simulink model "Closed_Loop_Model"  (R2020a)
settings: Solver=VariableStepAuto  StartTime=0.0  StopTime=inf  RelTol=1e-3
libraries: vrlib x9, simulink x7, visionsinks x1
settings Model: Creator=Jeffrey  LastModifiedBy=seanchai

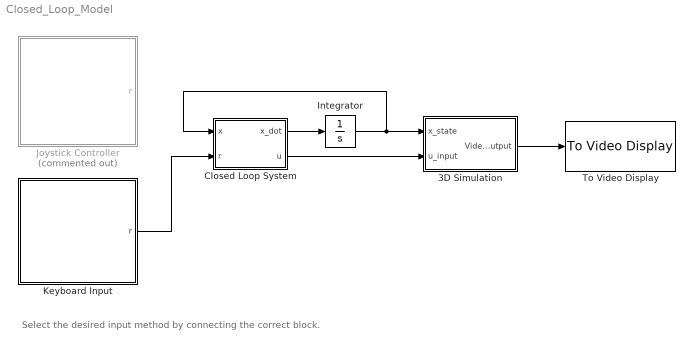
== system Closed_Loop_Model ==
  note: Select the desired input method by connecting the correct block.
  3D Simulation : Subsystem
  Closed Loop System : MATLAB Function  TreatAsAtomicUnit=on
  Integrator : Integrator  InitialCondition=[0; 0; 1; 0; 0; 0; 0; 0; 0; 0; 0; 0]
  Joystick Controller : Subsystem  Commented=on
  Keyboard Input : Subsystem
  To Video Display : visionsinks/To Video Display  windowSizeMode=Normal  openAtMdlStart=on  fullScreen=off  videoWindowX=577  videoWindowY=310  saveWindowSize=off  videoWindowWidth=640  videoWindowHeight=399  inputColorFormat=RGB  inputType=Obsolete  imagePorts=One multidimensional signal  OutputDevice=On-screen video monitor  dataOrg=Column-major  isWindowOpen=off
  wires:
  Integrator/1 -> 3D Simulation/1(x_state), Closed Loop System/1(x)
  Closed Loop System/1(x_dot) -> Integrator/1
  Closed Loop System/2(u) -> 3D Simulation/2(u_input)
  3D Simulation/1(Video Output) -> To Video Display/1
  Keyboard Input/1(r) -> Closed Loop System/2(r)

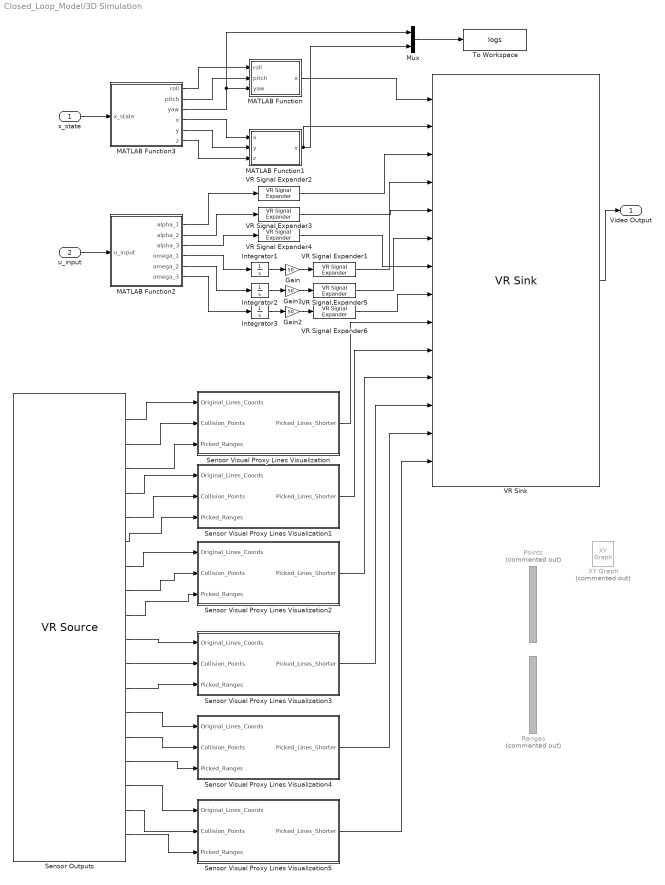
== system Closed_Loop_Model/3D Simulation ==
  x_state : Inport
  u_input : Inport  Port=2
  Gain : Gain  Gain=50
  Gain1 : Gain  Gain=50
  Gain2 : Gain  Gain=50
  Integrator1 : Integrator
  Integrator2 : Integrator
  Integrator3 : Integrator
  MATLAB Function : MATLAB Function  TreatAsAtomicUnit=on
  MATLAB Function1 : MATLAB Function  TreatAsAtomicUnit=on
  MATLAB Function2 : MATLAB Function  TreatAsAtomicUnit=on
  MATLAB Function3 : MATLAB Function  TreatAsAtomicUnit=on
  Mux : Mux  Inputs=2
  Points : Mux  Commented=on  Inputs=6
  Ranges : Mux  Commented=on  Inputs=6
  Sensor Outputs : vrlib/VR Source  InstantiateOnLoad=on  SampleTime=0.1  ViewEnable=on  RemoteChange=off  RemoteView=off  FieldsRead=Points_0006.point.61.3.1.double#PickSensor_0006.pickedPoint.60.3.1.double#PickSensor_0006.pickedRange.60.1.1.double#Points_0005.point.61.3.1.double#PickSensor_0005.pickedPoint.60.3.1.double#PickSensor_0005.pickedRange.60.1.1.double#Points_0004.point.61.3.1.double#PickSensor_0004.pickedPoint.60.3.1.double#PickSensor_0004.pickedRange.60.1.1.double#Points_0003.point.61.3.1.double#PickSensor_0003.pickedPoint.60.3.1.double#PickSensor_0003.pickedRange.60.1.1.double#Points_0002.point.61.3.1.double#PickSensor_0002.pickedPoint.60.3.1.double#PickSensor_0002.pickedRange.60.1.1.double#Points_0001.point.61.3.1.double#PickSensor_0001.pickedPoint.60.3.1.double#PickSensor_0001.pickedRange.60.1.1.double  WorldFileName=3DModel/3DModelTemplate  WorldDescription=Autonomous Airship  AutoView=on  VideoDimensions=[]  AllowVariableSize=on  FigureProperties="{'Position', 'Name', 'Viewpoint', 'CameraBound', 'CameraDirection', 'CameraPosition', 'CameraUpVector', 'ZoomFactor', 'Antialiasing', 'Headlight', 'Lighting', 'NavPanel', 'Sound', 'StatusBar', 'Stereo3D', 'Stereo3DCameraOffset', 'Stereo3DHIT', 'ToolBar', 'Textures', 'Transparency', 'Triad', 'Wireframe', 'NavZones', 'NavMode', 'NavSpeed', 'CaptureFileFormat', 'CaptureFileName', 'Record2DCompressMethod', 'Record2DCompressQuality', 'Record2D', 'Record2DFileName', 'Record2DFPS'; [1.3800000000000000e+02   1.0400000000000000e+02   5.7600000000000000e+02   3.5000000000000000e+02], 'Autonomous Airship', 'View from the Top', 'on', [0.0000000000000000e+00   0.0000000000000000e+00  -1.0000000000000000e+00], [0.0000000000000000e+00   0.0000000000000000e+00   0.0000000000000000e+00], [0.0000000000000000e+00   1.0000000000000000e+00   0.0000000000000000e+00], [1.0000000000000000e+00], 'on', 'on', 'on', 'halfbar', 'on', 'on', 'off', [1.0000000149011612e-01], [0.0000000000000000e+00], 'on', 'on', 'on', 'none', 'off', 'on', 'fly', 'normal', 'tif', '%f_anim_%n.tif', 'auto', [7.5000000000000000e+01], 'off', '%f_anim_%n.avi', 'auto'}"
      settings: SourceProductBaseCode=SL
  Sensor Visual Proxy Lines Visualization : Subsystem
  Sensor Visual Proxy Lines Visualization1 : Subsystem
  Sensor Visual Proxy Lines Visualization2 : Subsystem
  Sensor Visual Proxy Lines Visualization3 : Subsystem
  Sensor Visual Proxy Lines Visualization4 : Subsystem
  Sensor Visual Proxy Lines Visualization5 : Subsystem
  To Workspace : ToWorkspace  VariableName=logs  SampleTime=-1
      settings: Save2DSignal=2-D array (concatenate along first dimension)
  VR Signal Expander{1..6} (6 alike) : vrlib/VR Signal Expander  outwidth=4  outidx=[4]
  VR Sink : vrlib/VR Sink  InstantiateOnLoad=on  SampleTime=0.1  ViewEnable=on  RemoteChange=off  RemoteView=off  FieldsWritten=Airship.rotation.4.1.1.double#Airship.translation.3.1.1.double#Motor001.rotation.4.1.1.double#Prop001.rotation.4.1.1.double#Motor002.rotation.4.1.1.double#Prop002.rotation.4.1.1.double#Motor003.rotation.4.1.1.double#Prop003.rotation.4.1.1.double#Visual_Points_0006.point.3.-1.1.double#Visual_Points_0005.point.3.-1.1.double#Visual_Points_0004.point.3.-1.1.double#Visual_Points_0003.point.3.-1.1.double#Visual_Points_0002.point.3.-1.1.double#Visual_Points_0001.point.3.-1.1.double  WorldFileName=3DModel/3DModelTemplate.x3d  WorldDescription=Autonomous Airship  AutoView=on  VideoDimensions=[400 640]  AllowVariableSize=off  FigureProperties="{'Position', 'Name', 'Viewpoint', 'CameraBound', 'CameraDirection', 'CameraPosition', 'CameraUpVector', 'ZoomFactor', 'Antialiasing', 'Headlight', 'Lighting', 'NavPanel', 'Sound', 'StatusBar', 'Stereo3D', 'Stereo3DCameraOffset', 'Stereo3DHIT', 'ToolBar', 'Textures', 'Transparency', 'Triad', 'Wireframe', 'NavZones', 'NavMode', 'NavSpeed', 'CaptureFileFormat', 'CaptureFileName', 'Record2DCompressMethod', 'Record2DCompressQuality', 'Record2D', 'Record2DFileName', 'Record2DFPS'; [5.0000000000000000e+00   9.5000000000000000e+01   5.7600000000000000e+02   3.5000000000000000e+02], 'Autonomous Airship', 'View from the Top', 'on', [-6.0928554571654234e-02  -3.0894106635612190e-01  -9.4912756189910374e-01], [-1.3366649406455859e+00   3.5008055805870580e-01  -4.6890079737670746e+01], [-1.4625128619556730e-02   9.5106843948065223e-01  -3.0863397259001091e-01], [1.0000000000000000e+00], 'off', 'on', 'on', 'halfbar', 'on', 'on', 'off', [1.0000000149011612e-01], [0.0000000000000000e+00], 'on', 'on', 'on', 'none', 'off', 'on', 'fly', 'normal', 'tif', '%f_anim_%n.tif', 'auto', [7.5000000000000000e+01], 'off', '%f_anim_%n.avi', 'auto'; [5.8600000000000000e+02   6.0000000000000000e+01   6.4000000000000000e+02   4.0000000000000000e+02], 'Autonomous Airship', 'SensorCam ', 'on', [0.0000000000000000e+00   0.0000000000000000e+00  -1.0000000000000000e+00], [0.0000000000000000e+00   0.0000000000000000e+00   0.0000000000000000e+00], [0.0000000000000000e+00   1.0000000000000000e+00   0.0000000000000000e+00], [1.0000000000000000e+00], 'on', 'on', 'on', 'none', 'on', 'off', 'off', [1.0000000149011612e-01], [0.0000000000000000e+00], 'off', 'on', 'on', 'none', 'off', 'off', 'fly', 'normal', 'tif', '%f_anim_%n.tif', 'auto', [7.5000000000000000e+01], 'off', '***video***', 'auto'}"
  XY Graph : simulink/Sinks/XY Graph  Commented=on  xmin=-1  xmax=1  ymin=-1  ymax=1  st=-1
  Video Output : Outport
  wires:
  MATLAB Function3/5(y) -> MATLAB Function1/2(y)
  x_state/1 -> MATLAB Function3/1(x_state)
  MATLAB Function3/4(x) -> MATLAB Function1/1(x)
  MATLAB Function2/2(alpha_2) -> VR Signal Expander3/1
  MATLAB Function2/3(alpha_3) -> VR Signal Expander4/1
  MATLAB Function2/1(alpha_1) -> VR Signal Expander2/1
  MATLAB Function3/1(roll) -> MATLAB Function/1(roll)
  MATLAB Function2/5(omega_2) -> Integrator2/1
  Gain2/1 -> VR Signal Expander6/1
  Gain/1 -> VR Signal Expander1/1
  MATLAB Function3/6(z) -> MATLAB Function1/3(z)
  Gain1/1 -> VR Signal Expander5/1
  Integrator1/1 -> Gain/1
  MATLAB Function3/2(pitch) -> MATLAB Function/2(pitch)
  Integrator2/1 -> Gain1/1
  Integrator3/1 -> Gain2/1
  MATLAB Function2/6(omega_3) -> Integrator3/1
  VR Sink/1 -> Video Output/1
  MATLAB Function2/4(omega_1) -> Integrator1/1
  u_input/1 -> MATLAB Function2/1(u_input)
  Mux/1 -> To Workspace/1
  MATLAB Function3/3(yaw) -> Mux/1, MATLAB Function/3(yaw)
  MATLAB Function1/1(v) -> Mux/2, VR Sink/2
  Sensor Outputs/1 -> Sensor Visual Proxy Lines Visualization/1(Original_Lines_Coords)
  Sensor Outputs/2 -> Sensor Visual Proxy Lines Visualization/2(Collision_Points)
  Sensor Outputs/3 -> Sensor Visual Proxy Lines Visualization/3(Picked_Ranges)
  MATLAB Function/1(x) -> VR Sink/1
  VR Signal Expander2/1 -> VR Sink/3
  VR Signal Expander1/1 -> VR Sink/4
  VR Signal Expander3/1 -> VR Sink/5
  VR Signal Expander5/1 -> VR Sink/6
  VR Signal Expander4/1 -> VR Sink/7
  VR Signal Expander6/1 -> VR Sink/8
  Sensor Outputs/4 -> Sensor Visual Proxy Lines Visualization1/1(Original_Lines_Coords)
  Sensor Outputs/5 -> Sensor Visual Proxy Lines Visualization1/2(Collision_Points)
  Sensor Outputs/6 -> Sensor Visual Proxy Lines Visualization1/3(Picked_Ranges)
  Sensor Outputs/8 -> Sensor Visual Proxy Lines Visualization2/2(Collision_Points)
  Sensor Outputs/9 -> Sensor Visual Proxy Lines Visualization2/3(Picked_Ranges)
  Sensor Outputs/10 -> Sensor Visual Proxy Lines Visualization3/1(Original_Lines_Coords)
  Sensor Outputs/11 -> Sensor Visual Proxy Lines Visualization3/2(Collision_Points)
  Sensor Outputs/12 -> Sensor Visual Proxy Lines Visualization3/3(Picked_Ranges)
  Sensor Outputs/13 -> Sensor Visual Proxy Lines Visualization4/1(Original_Lines_Coords)
  Sensor Outputs/14 -> Sensor Visual Proxy Lines Visualization4/2(Collision_Points)
  Sensor Outputs/15 -> Sensor Visual Proxy Lines Visualization4/3(Picked_Ranges)
  Sensor Outputs/16 -> Sensor Visual Proxy Lines Visualization5/1(Original_Lines_Coords)
  Sensor Outputs/17 -> Sensor Visual Proxy Lines Visualization5/2(Collision_Points)
  Sensor Outputs/18 -> Sensor Visual Proxy Lines Visualization5/3(Picked_Ranges)
  Sensor Outputs/7 -> Sensor Visual Proxy Lines Visualization2/1(Original_Lines_Coords)
  Sensor Visual Proxy Lines Visualization/1(Picked_Lines_Shorter) -> VR Sink/9
  Sensor Visual Proxy Lines Visualization1/1(Picked_Lines_Shorter) -> VR Sink/10
  Sensor Visual Proxy Lines Visualization2/1(Picked_Lines_Shorter) -> VR Sink/11
  Sensor Visual Proxy Lines Visualization3/1(Picked_Lines_Shorter) -> VR Sink/12
  Sensor Visual Proxy Lines Visualization4/1(Picked_Lines_Shorter) -> VR Sink/13
  Sensor Visual Proxy Lines Visualization5/1(Picked_Lines_Shorter) -> VR Sink/14

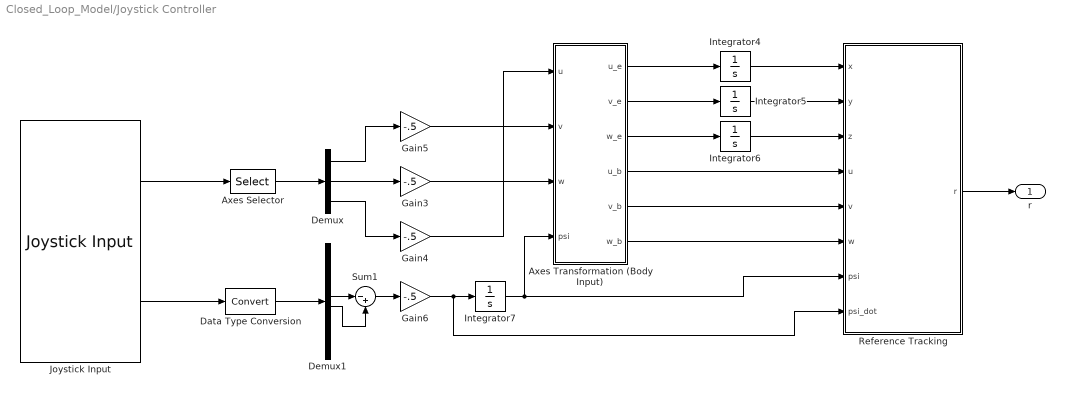
== system Closed_Loop_Model/Joystick Controller ==
  Axes Selector : Selector  InputPortWidth=5  IndexOptions=Index vector (dialog)  Indices=[1 3 2]  OutputSizes=1
      settings: AttributesFormatString=(Joystick - dependent)
  Axes Transformation (Body Input) : MATLAB Function  TreatAsAtomicUnit=on
  Data Type Conversion : DataTypeConversion
  Demux : Demux  Outputs=3
  Demux1 : Demux  Outputs=10
  Gain{3..6} (4 alike) : Gain  Gain=-.5
  Integrator4 : Integrator
  Integrator5 : Integrator
  Integrator6 : Integrator  InitialCondition=1
  Integrator7 : Integrator
  Joystick Input : vrlib/Joystick Input  joyid=1  adjustports=on  forcefeed=off
  Reference Tracking : MATLAB Function  TreatAsAtomicUnit=on
  Sum1 : Sum  Inputs=|-+
  r : Outport
  wires:
  Gain3/1 -> Axes Transformation (Body Input)/3(w)
  Demux/2 -> Gain3/1
  Gain5/1 -> Axes Transformation (Body Input)/2(v)
  Joystick Input/1 -> Axes Selector/1
  Axes Selector/1 -> Demux/1
  Joystick Input/2 -> Data Type Conversion/1
  Demux1/5 -> Sum1/1
  Demux/3 -> Gain4/1
  Gain4/1 -> Axes Transformation (Body Input)/1(u)
  Demux/1 -> Gain5/1
  Sum1/1 -> Gain6/1
  Data Type Conversion/1 -> Demux1/1
  Demux1/6 -> Sum1/2
  Integrator5/1 -> Reference Tracking/2(y)
  Integrator6/1 -> Reference Tracking/3(z)
  Integrator4/1 -> Reference Tracking/1(x)
  Integrator7/1 -> Reference Tracking/7(psi), Axes Transformation (Body Input)/4(psi)
  Gain6/1 -> Reference Tracking/8(psi_dot), Integrator7/1
  Axes Transformation (Body Input)/4(u_b) -> Reference Tracking/4(u)
  Axes Transformation (Body Input)/5(v_b) -> Reference Tracking/5(v)
  Axes Transformation (Body Input)/6(w_b) -> Reference Tracking/6(w)
  Axes Transformation (Body Input)/3(w_e) -> Integrator6/1
  Axes Transformation (Body Input)/2(v_e) -> Integrator5/1
  Axes Transformation (Body Input)/1(u_e) -> Integrator4/1
  Reference Tracking/1(r) -> r/1

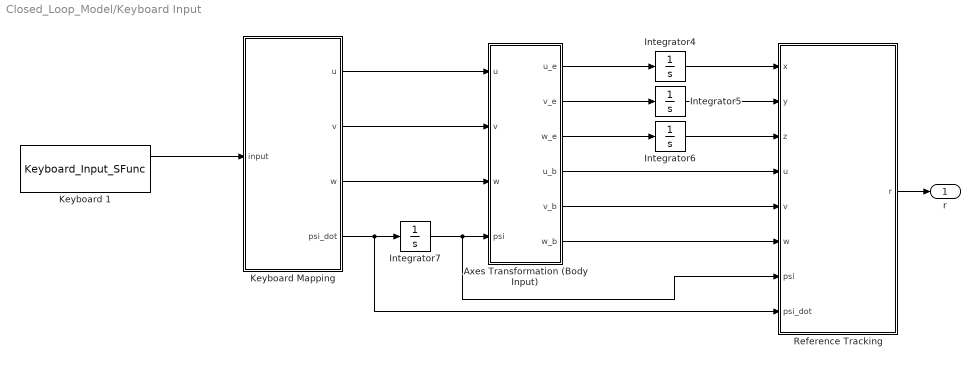
== system Closed_Loop_Model/Keyboard Input ==
  Axes Transformation (Body Input) : MATLAB Function  TreatAsAtomicUnit=on
  Integrator4 : Integrator
  Integrator5 : Integrator
  Integrator6 : Integrator  InitialCondition=1
  Integrator7 : Integrator
  Keyboard 1 : M-S-Function  FunctionName=Keyboard_Input_SFunc  mask(Keyboard Input){}
      mask help: Keyboard Input
      mask Display: fprintf('Keyboard');
  Keyboard Mapping : MATLAB Function  TreatAsAtomicUnit=on
  Reference Tracking : MATLAB Function  TreatAsAtomicUnit=on
  r : Outport
  wires:
  Axes Transformation (Body Input)/5(v_b) -> Reference Tracking/5(v)
  Integrator5/1 -> Reference Tracking/2(y)
  Axes Transformation (Body Input)/6(w_b) -> Reference Tracking/6(w)
  Axes Transformation (Body Input)/4(u_b) -> Reference Tracking/4(u)
  Integrator6/1 -> Reference Tracking/3(z)
  Integrator4/1 -> Reference Tracking/1(x)
  Axes Transformation (Body Input)/1(u_e) -> Integrator4/1
  Axes Transformation (Body Input)/3(w_e) -> Integrator6/1
  Axes Transformation (Body Input)/2(v_e) -> Integrator5/1
  Integrator7/1 -> Reference Tracking/7(psi), Axes Transformation (Body Input)/4(psi)
  Reference Tracking/1(r) -> r/1
  Keyboard 1/1 -> Keyboard Mapping/1(input)
  Keyboard Mapping/1(u) -> Axes Transformation (Body Input)/1(u)
  Keyboard Mapping/2(v) -> Axes Transformation (Body Input)/2(v)
  Keyboard Mapping/3(w) -> Axes Transformation (Body Input)/3(w)
  Keyboard Mapping/4(psi_dot) -> Integrator7/1, Reference Tracking/8(psi_dot)

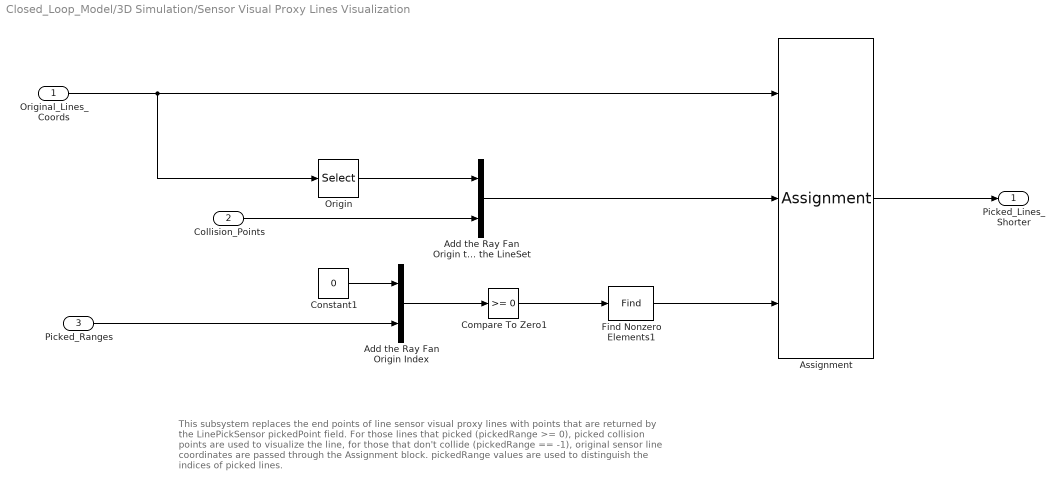
== system Closed_Loop_Model/3D Simulation/Sensor Visual Proxy Lines Visualization ==
  note: This subsystem replaces the end points of line sensor visual proxy lines with points that are returned by the LinePickSensor pickedPoint field.
      | For those lines that picked (pickedRange >= 0), picked collision points are used to visualize the line, for those that don't collide (pickedRange == -1),
      | original sensor line coordinates are passed through the Assignment block. pickedRange values are used to distinguish the indices of picked lines.
  Original_Lines_Coords : Inport
  Collision_Points : Inport  Port=2
  Picked_Ranges : Inport  Port=3
  Add the Ray Fan Origin Index : Concatenate  Mode=Multidimensional array
  Add the Ray Fan Origin to the LineSet : Concatenate  Mode=Multidimensional array
  Assignment : Assignment  NumberOfDimensions=2  DiagnosticForDimensions=Warning  IndexOptions=Index vector (port),Assign all  Indices=1,1  OutputSizes=1,1
  Compare To Zero1 : simulink/Logic and Bit Operations/Compare To Zero  relop=>=  OutDataTypeStr=boolean
  Constant1 : Constant  Value=0
  Find Nonzero Elements1 : Find  NumberOfInputDimensions=3
  Origin : Selector  NumberOfDimensions=2  InputPortWidth=3  IndexOptions=Index vector (dialog),Index vector (dialog)  Indices=1,[1 2 3]  OutputSizes=1,1
  Picked_Lines_Shorter : Outport  VectorParamsAs1DForOutWhenUnconnected=off
  wires:
  Collision_Points/1 -> Add the Ray Fan Origin to the LineSet/2
  Assignment/1 -> Picked_Lines_Shorter/1
  Origin/1 -> Add the Ray Fan Origin to the LineSet/1
  Original_Lines_Coords/1 -> Assignment/1, Origin/1
  Constant1/1 -> Add the Ray Fan Origin Index/1
  Picked_Ranges/1 -> Add the Ray Fan Origin Index/2
  Find Nonzero Elements1/1 -> Assignment/3
  Add the Ray Fan Origin to the LineSet/1 -> Assignment/2
  Add the Ray Fan Origin Index/1 -> Compare To Zero1/1
  Compare To Zero1/1 -> Find Nonzero Elements1/1

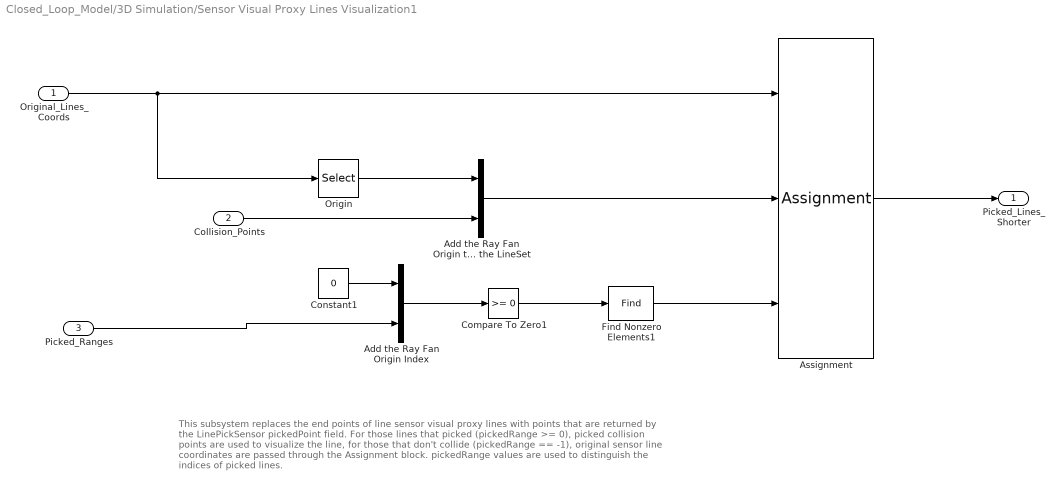
== system Closed_Loop_Model/3D Simulation/Sensor Visual Proxy Lines Visualization1 ==
  note: This subsystem replaces the end points of line sensor visual proxy lines with points that are returned by the LinePickSensor pickedPoint field.
      | For those lines that picked (pickedRange >= 0), picked collision points are used to visualize the line, for those that don't collide (pickedRange == -1),
      | original sensor line coordinates are passed through the Assignment block. pickedRange values are used to distinguish the indices of picked lines.
  Original_Lines_Coords : Inport
  Collision_Points : Inport  Port=2
  Picked_Ranges : Inport  Port=3
  Add the Ray Fan Origin Index : Concatenate  Mode=Multidimensional array
  Add the Ray Fan Origin to the LineSet : Concatenate  Mode=Multidimensional array
  Assignment : Assignment  NumberOfDimensions=2  DiagnosticForDimensions=Warning  IndexOptions=Index vector (port),Assign all  Indices=1,1  OutputSizes=1,1
  Compare To Zero1 : simulink/Logic and Bit Operations/Compare To Zero  relop=>=  OutDataTypeStr=boolean
  Constant1 : Constant  Value=0
  Find Nonzero Elements1 : Find  NumberOfInputDimensions=3
  Origin : Selector  NumberOfDimensions=2  InputPortWidth=3  IndexOptions=Index vector (dialog),Index vector (dialog)  Indices=1,[1 2 3]  OutputSizes=1,1
  Picked_Lines_Shorter : Outport  VectorParamsAs1DForOutWhenUnconnected=off
  wires:
  Collision_Points/1 -> Add the Ray Fan Origin to the LineSet/2
  Assignment/1 -> Picked_Lines_Shorter/1
  Origin/1 -> Add the Ray Fan Origin to the LineSet/1
  Original_Lines_Coords/1 -> Assignment/1, Origin/1
  Compare To Zero1/1 -> Find Nonzero Elements1/1
  Add the Ray Fan Origin Index/1 -> Compare To Zero1/1
  Constant1/1 -> Add the Ray Fan Origin Index/1
  Picked_Ranges/1 -> Add the Ray Fan Origin Index/2
  Find Nonzero Elements1/1 -> Assignment/3
  Add the Ray Fan Origin to the LineSet/1 -> Assignment/2

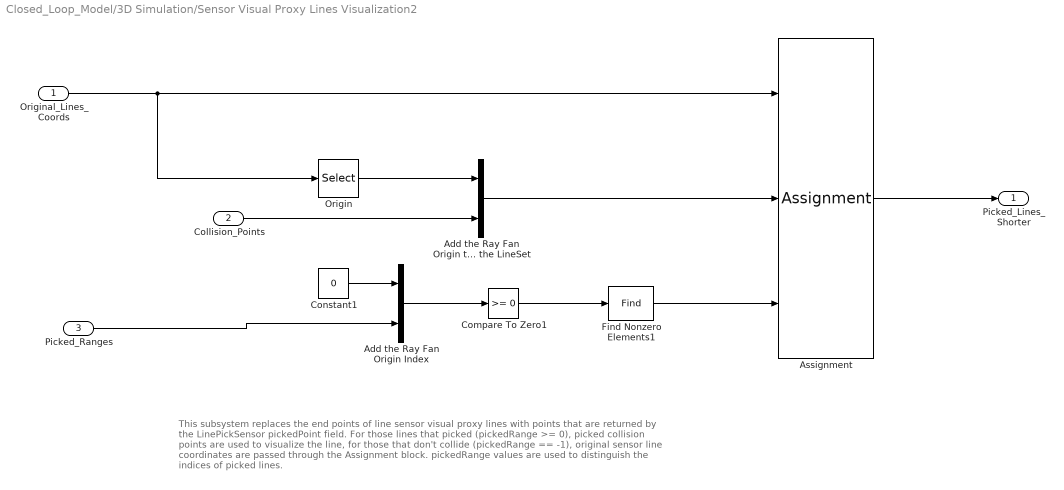
== system Closed_Loop_Model/3D Simulation/Sensor Visual Proxy Lines Visualization2 ==
  note: This subsystem replaces the end points of line sensor visual proxy lines with points that are returned by the LinePickSensor pickedPoint field.
      | For those lines that picked (pickedRange >= 0), picked collision points are used to visualize the line, for those that don't collide (pickedRange == -1),
      | original sensor line coordinates are passed through the Assignment block. pickedRange values are used to distinguish the indices of picked lines.
  Original_Lines_Coords : Inport
  Collision_Points : Inport  Port=2
  Picked_Ranges : Inport  Port=3
  Add the Ray Fan Origin Index : Concatenate  Mode=Multidimensional array
  Add the Ray Fan Origin to the LineSet : Concatenate  Mode=Multidimensional array
  Assignment : Assignment  NumberOfDimensions=2  DiagnosticForDimensions=Warning  IndexOptions=Index vector (port),Assign all  Indices=1,1  OutputSizes=1,1
  Compare To Zero1 : simulink/Logic and Bit Operations/Compare To Zero  relop=>=  OutDataTypeStr=boolean
  Constant1 : Constant  Value=0
  Find Nonzero Elements1 : Find  NumberOfInputDimensions=3
  Origin : Selector  NumberOfDimensions=2  InputPortWidth=3  IndexOptions=Index vector (dialog),Index vector (dialog)  Indices=1,[1 2 3]  OutputSizes=1,1
  Picked_Lines_Shorter : Outport  VectorParamsAs1DForOutWhenUnconnected=off
  wires:
  Collision_Points/1 -> Add the Ray Fan Origin to the LineSet/2
  Assignment/1 -> Picked_Lines_Shorter/1
  Origin/1 -> Add the Ray Fan Origin to the LineSet/1
  Original_Lines_Coords/1 -> Assignment/1, Origin/1
  Compare To Zero1/1 -> Find Nonzero Elements1/1
  Add the Ray Fan Origin Index/1 -> Compare To Zero1/1
  Constant1/1 -> Add the Ray Fan Origin Index/1
  Picked_Ranges/1 -> Add the Ray Fan Origin Index/2
  Find Nonzero Elements1/1 -> Assignment/3
  Add the Ray Fan Origin to the LineSet/1 -> Assignment/2

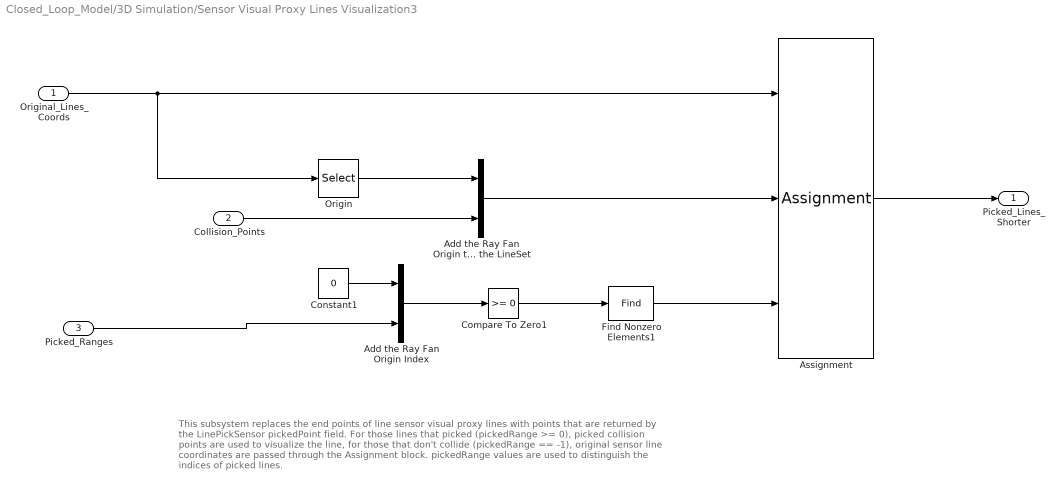
== system Closed_Loop_Model/3D Simulation/Sensor Visual Proxy Lines Visualization3 ==
  note: This subsystem replaces the end points of line sensor visual proxy lines with points that are returned by the LinePickSensor pickedPoint field.
      | For those lines that picked (pickedRange >= 0), picked collision points are used to visualize the line, for those that don't collide (pickedRange == -1),
      | original sensor line coordinates are passed through the Assignment block. pickedRange values are used to distinguish the indices of picked lines.
  Original_Lines_Coords : Inport
  Collision_Points : Inport  Port=2
  Picked_Ranges : Inport  Port=3
  Add the Ray Fan Origin Index : Concatenate  Mode=Multidimensional array
  Add the Ray Fan Origin to the LineSet : Concatenate  Mode=Multidimensional array
  Assignment : Assignment  NumberOfDimensions=2  DiagnosticForDimensions=Warning  IndexOptions=Index vector (port),Assign all  Indices=1,1  OutputSizes=1,1
  Compare To Zero1 : simulink/Logic and Bit Operations/Compare To Zero  relop=>=  OutDataTypeStr=boolean
  Constant1 : Constant  Value=0
  Find Nonzero Elements1 : Find  NumberOfInputDimensions=3
  Origin : Selector  NumberOfDimensions=2  InputPortWidth=3  IndexOptions=Index vector (dialog),Index vector (dialog)  Indices=1,[1 2 3]  OutputSizes=1,1
  Picked_Lines_Shorter : Outport  VectorParamsAs1DForOutWhenUnconnected=off
  wires:
  Collision_Points/1 -> Add the Ray Fan Origin to the LineSet/2
  Assignment/1 -> Picked_Lines_Shorter/1
  Origin/1 -> Add the Ray Fan Origin to the LineSet/1
  Original_Lines_Coords/1 -> Assignment/1, Origin/1
  Compare To Zero1/1 -> Find Nonzero Elements1/1
  Add the Ray Fan Origin Index/1 -> Compare To Zero1/1
  Constant1/1 -> Add the Ray Fan Origin Index/1
  Picked_Ranges/1 -> Add the Ray Fan Origin Index/2
  Find Nonzero Elements1/1 -> Assignment/3
  Add the Ray Fan Origin to the LineSet/1 -> Assignment/2

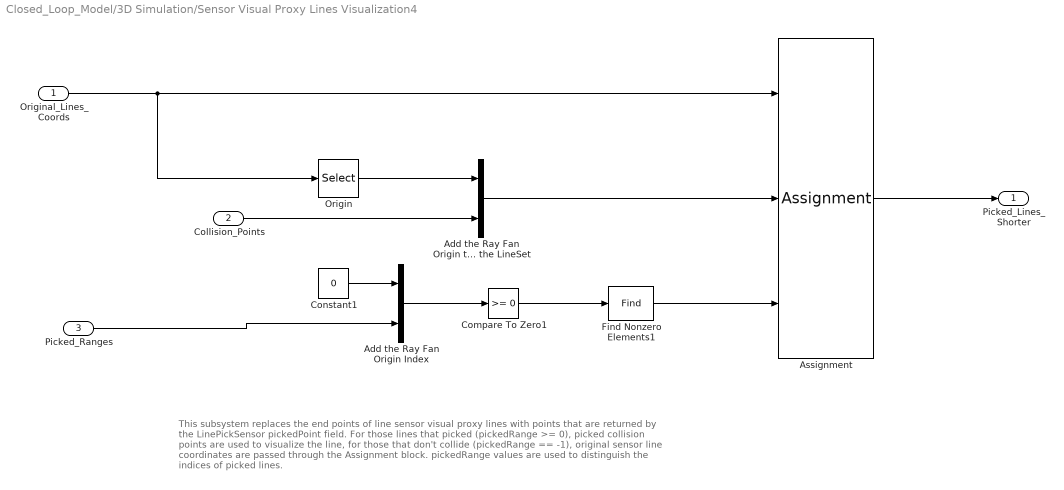
== system Closed_Loop_Model/3D Simulation/Sensor Visual Proxy Lines Visualization4 ==
  note: This subsystem replaces the end points of line sensor visual proxy lines with points that are returned by the LinePickSensor pickedPoint field.
      | For those lines that picked (pickedRange >= 0), picked collision points are used to visualize the line, for those that don't collide (pickedRange == -1),
      | original sensor line coordinates are passed through the Assignment block. pickedRange values are used to distinguish the indices of picked lines.
  Original_Lines_Coords : Inport
  Collision_Points : Inport  Port=2
  Picked_Ranges : Inport  Port=3
  Add the Ray Fan Origin Index : Concatenate  Mode=Multidimensional array
  Add the Ray Fan Origin to the LineSet : Concatenate  Mode=Multidimensional array
  Assignment : Assignment  NumberOfDimensions=2  DiagnosticForDimensions=Warning  IndexOptions=Index vector (port),Assign all  Indices=1,1  OutputSizes=1,1
  Compare To Zero1 : simulink/Logic and Bit Operations/Compare To Zero  relop=>=  OutDataTypeStr=boolean
  Constant1 : Constant  Value=0
  Find Nonzero Elements1 : Find  NumberOfInputDimensions=3
  Origin : Selector  NumberOfDimensions=2  InputPortWidth=3  IndexOptions=Index vector (dialog),Index vector (dialog)  Indices=1,[1 2 3]  OutputSizes=1,1
  Picked_Lines_Shorter : Outport  VectorParamsAs1DForOutWhenUnconnected=off
  wires:
  Collision_Points/1 -> Add the Ray Fan Origin to the LineSet/2
  Assignment/1 -> Picked_Lines_Shorter/1
  Origin/1 -> Add the Ray Fan Origin to the LineSet/1
  Original_Lines_Coords/1 -> Assignment/1, Origin/1
  Compare To Zero1/1 -> Find Nonzero Elements1/1
  Add the Ray Fan Origin Index/1 -> Compare To Zero1/1
  Constant1/1 -> Add the Ray Fan Origin Index/1
  Picked_Ranges/1 -> Add the Ray Fan Origin Index/2
  Find Nonzero Elements1/1 -> Assignment/3
  Add the Ray Fan Origin to the LineSet/1 -> Assignment/2

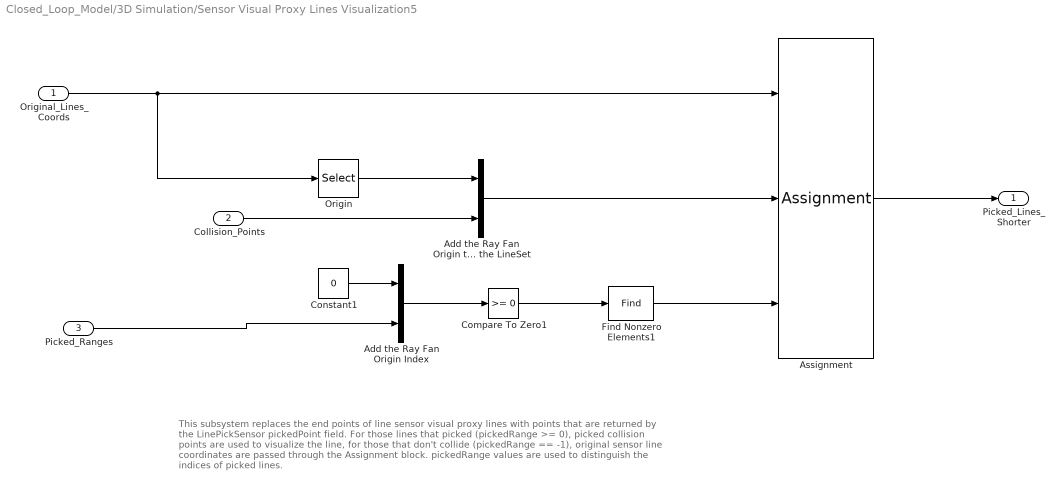
== system Closed_Loop_Model/3D Simulation/Sensor Visual Proxy Lines Visualization5 ==
  note: This subsystem replaces the end points of line sensor visual proxy lines with points that are returned by the LinePickSensor pickedPoint field.
      | For those lines that picked (pickedRange >= 0), picked collision points are used to visualize the line, for those that don't collide (pickedRange == -1),
      | original sensor line coordinates are passed through the Assignment block. pickedRange values are used to distinguish the indices of picked lines.
  Original_Lines_Coords : Inport
  Collision_Points : Inport  Port=2
  Picked_Ranges : Inport  Port=3
  Add the Ray Fan Origin Index : Concatenate  Mode=Multidimensional array
  Add the Ray Fan Origin to the LineSet : Concatenate  Mode=Multidimensional array
  Assignment : Assignment  NumberOfDimensions=2  DiagnosticForDimensions=Warning  IndexOptions=Index vector (port),Assign all  Indices=1,1  OutputSizes=1,1
  Compare To Zero1 : simulink/Logic and Bit Operations/Compare To Zero  relop=>=  OutDataTypeStr=boolean
  Constant1 : Constant  Value=0
  Find Nonzero Elements1 : Find  NumberOfInputDimensions=3
  Origin : Selector  NumberOfDimensions=2  InputPortWidth=3  IndexOptions=Index vector (dialog),Index vector (dialog)  Indices=1,[1 2 3]  OutputSizes=1,1
  Picked_Lines_Shorter : Outport  VectorParamsAs1DForOutWhenUnconnected=off
  wires:
  Collision_Points/1 -> Add the Ray Fan Origin to the LineSet/2
  Assignment/1 -> Picked_Lines_Shorter/1
  Origin/1 -> Add the Ray Fan Origin to the LineSet/1
  Original_Lines_Coords/1 -> Assignment/1, Origin/1
  Compare To Zero1/1 -> Find Nonzero Elements1/1
  Add the Ray Fan Origin Index/1 -> Compare To Zero1/1
  Constant1/1 -> Add the Ray Fan Origin Index/1
  Picked_Ranges/1 -> Add the Ray Fan Origin Index/2
  Find Nonzero Elements1/1 -> Assignment/3
  Add the Ray Fan Origin to the LineSet/1 -> Assignment/2

== matlab function Closed_Loop_Model/Keyboard Input/Keyboard Mapping ==
  data: input input; u output; v output; w output; psi_dot output
function [u,v,w,psi_dot] = fcn(input)
% Implements Blocking Keyboard Input
%WASD Translation Control
% SHIFT CTRL Altitude Control
%QE Yaw Control
%SPACE to Stop

u=0;
v=0;
w=0;
psi_dot=0;

%SPACE
if input == 32
    u=0; v=0; w=0; psi_dot=0;
end

%Translation - x
if input == 119
    u = 0.5;
elseif input == 115
    u = -0.5;
end

%Translation - y
if input == 100
    v = -0.5;
elseif input == 97
    v = 0.5;
end

%Altitude
if input == 114
    w = 0.5;
elseif input == 102
    w = -0.5;
end

%Yaw
if input == 101
    psi_dot = -0.25;
elseif input == 113
    psi_dot = 0.25;
end

== matlab function Closed_Loop_Model/Keyboard Input/Axes Transformation (Body Input) ==
  data: u input; u_e output; v input; w input; v_e output; w_e output; psi input; u_b output; v_b output; w_b output
function [u_e,v_e,w_e,u_b,v_b,w_b] = fcn(u, v, w, psi)

%rotating uvw vector (assume input u v w in body frame)
a=0; b=0; c=psi;
T_roll = [ 1, 0      , 0    ;
         0, cos(a) , sin(a) ;
         0, -sin(a), cos(a) ];
     
T_pitch = [cos(b),0,-sin(b) ;
        0     ,1,0       ;
        sin(b),0,cos(b)  ];
    
T_yaw = [cos(c) ,sin(c),0;
        -sin(c),cos(c),0;
        0      ,0     ,1];

T_BE = T_roll * T_pitch * T_yaw;

V_e = T_BE^-1 * [u;v;w];

u_e = V_e(1);
v_e = V_e(2);
w_e = V_e(3);

u_b = u;
v_b = v;
w_b = w;

== matlab function Closed_Loop_Model/Keyboard Input/Reference Tracking ==
  data: x input; y input; z input; r output; u input; v input; w input; psi input; psi_dot input
function r = fcn(x,y,z,u,v,w,psi,psi_dot)

r = zeros(12,1);
% reference output
r(1) = x;
r(2) = y;
r(3) = z;
r(4) = u;
r(5) = v;
r(6) = w;
r(9) = psi;
r(12) = psi_dot;

== matlab function Closed_Loop_Model/3D Simulation/MATLAB Function1 ==
  data: x input; v output; y input; z input
function v = fcn(x,y,z)

v = [x , z, -y];

== matlab function Closed_Loop_Model/3D Simulation/MATLAB Function ==
  data: roll input; x output; pitch input; yaw input
function x = fcn(roll,pitch,yaw) %local pitch and roll
a = -roll;
b = pitch;
c = -yaw;

T_roll = [ 1, 0      , 0    ;
         0, cos(a) , sin(a) ;
         0, -sin(a), cos(a) ];
     
T_pitch = [cos(b),0,-sin(b) ;
        0     ,1,0       ;
        sin(b),0,cos(b)  ];
    
T_yaw = [cos(c) ,sin(c),0;
        -sin(c),cos(c),0;
        0      ,0     ,1];


T_BE = T_roll * T_pitch * T_yaw;
        
        
v = rotationMatrixToVector (T_BE^-1);

x = [v(1),v(3),v(2), norm(v)];

== matlab function Closed_Loop_Model/Joystick Controller/Reference Tracking ==
  data: x input; y input; z input; r output; u input; v input; w input; psi input; psi_dot input
function r = fcn(x,y,z,u,v,w,psi,psi_dot)

r = zeros(12,1);
% reference output
r(1) = x;
r(2) = y;
r(3) = z;
r(4) = u;
r(5) = v;
r(6) = w;
r(9) = psi;
r(12) = psi_dot;

== matlab function Closed_Loop_Model/3D Simulation/MATLAB Function3 ==
  data: roll output; pitch output; yaw output; x output; x_state input; y output; z output
function [roll,pitch,yaw,x,y,z] = fcn(x_state)

x = x_state(1);
y = x_state(2);
z = x_state(3);
roll = x_state(7);
pitch = x_state(8);
yaw = x_state(9);

== matlab function Closed_Loop_Model/3D Simulation/MATLAB Function2 ==
  data: alpha_1 output; alpha_2 output; alpha_3 output; omega_1 output; u_input input; omega_2 output; omega_3 output
function [alpha_1,alpha_2,alpha_3,omega_1,omega_2,omega_3] = fcn(u_input)

omega_1 = u_input(1);
omega_2 = u_input(2);
omega_3 = u_input(3);
alpha_1 = u_input(4);
alpha_2 = u_input(5);
alpha_3 = u_input(6);

== matlab function Closed_Loop_Model/Closed Loop System ==
  data: x input; x_dot output; r input; u output
function [x_dot,u] = fcn(x,r)
A = [0,0,0,1,0,0,0,0,0,0,0,0;0,0,0,0,1,0,0,0,0,0,0,0;0,0,0,0,0,1,0,0,0,0,0,0;0,0,0,0,0,0,0,5.40600000000000,0,0,0,0;0,0,0,0,0,0,-5.40600000000000,0,0,0,0,0;0,0,0,0,0,0,0,0,0,0,0,0;0,0,0,0,0,0,0,0,0,1,0,0;0,0,0,0,0,0,0,0,0,0,1,0;0,0,0,0,0,0,0,0,0,0,0,1;0,0,0,0,0,0,0,0,0,0,0,0;0,0,0,0,0,0,0,0,0,0,0,0;0,0,0,0,0,0,0,0,0,0,0,0];
B = [0,0,0,0,0,0;0,0,0,0,0,0;0,0,0,0,0,0;0,0,0,0,2.59807621135332,-2.59807621135332;0,0,0,-3,1.50000000000000,1.50000000000000;1.20000000000000,1.20000000000000,1.20000000000000,0,0,0;0,0,0,0,0,0;0,0,0,0,0,0;0,0,0,0,0,0;0.625000000000000,-0.998797632095823,2.24879763209582,2.50000000000000,-6.60957346706593,-6.60957346706593;1.80000000000000,-0.900000000000000,-0.900000000000000,7.50000000000000,-2.45096189432334,-5.04903810567666;3.12500000000000,2.80024047358084,3.44975952641916,5,3.17808530658681,3.17808530658681];
C = [8.99321605918731e-06,0,0,0,0,0,0,0,0,0,0,0;2.21564316353217e-19,8.99321605918742e-06,0,0,0,0,0,0,0,0,0,0;0,0,1,0,0,0,0,0,0,0,0,0;0,0,0,1,0,0,0,0,0,0,0,0;0,0,0,0,1,0,0,0,0,0,0,0;0,0,0,0,0,1,0,0,0,0,0,0;0,0,0,0,0,0,0,0,1,0,0,0;0,0,0,0,0,0,0,0,0,1,0,0;0,0,0,0,0,0,0,0,0,0,1,0;0,0,0,0,0,0,0,0,0,0,0,1];
D = [0,0,0,0,0,0;0,0,0,0,0,0;0,0,0,0,0,0;0,0,0,0,0,0;0,0,0,0,0,0;0,0,0,0,0,0;0,0,0,0,0,0;0,0,0,0,0,0;0,0,0,0,0,0;0,0,0,0,0,0];
K = [-0.397441583161921,1.88832444607901,1.76916801580035,-0.495873279885801,2.39632253767234,2.12552937228456,-2.74521810854438,0.709348694221778,0.866553788130112,-0.0334752382522595,1.48248826385365,0.836775567257872;0.182607622717259,-1.45712014204255,2.34535206644118,0.201238674695816,-1.98013482185658,3.07333818528282,2.53529001380557,-0.570917695231242,0.630549955837904,-0.453145510174142,-0.732315097573767,0.482041889876711;0.491316108942495,-0.127744464173746,-0.226940860637152,0.596386348794549,-0.453751907350929,-0.399642523186977,3.66807301130215,-1.00942055374447,1.95172885644241,2.05851640916043,-1.84665184515622,2.09432411224338;-0.204972178169728,-1.52739351320494,-0.778121415793965,-0.154708017641559,-1.76688876592689,-0.985294996914921,1.38219254554613,2.36824233463773,1.65290490572560,0.0851515061825858,2.07501904405081,1.73567492229963;2.11161042060494,1.17518699442540,-0.562927488275802,2.23546874101000,1.75800173849048,-0.928983712584736,-5.10140531370422,0.693886856218595,1.01798554914721,-1.90194038249112,0.145738536909078,1.15021120006268;-2.25086449235886,0.762048301500732,-0.628892492647789,-2.50754852407902,1.28427063452888,-0.949814813671555,-4.51937850829551,-2.29965063799660,1.12865253765537,-1.66203430705188,-0.799768900154175,1.24684642040635];
u = K*(r-x);
x_dot = A*x+B*u;
%y=C*x

== matlab function Closed_Loop_Model/Joystick Controller/Axes Transformation (Body Input) ==
  data: u input; u_e output; v input; w input; v_e output; w_e output; psi input; u_b output; v_b output; w_b output
function [u_e,v_e,w_e,u_b,v_b,w_b] = fcn(u, v, w, psi)

%rotating uvw vector (assume input u v w in body frame)
a=0; b=0; c=psi;
T_roll = [ 1, 0      , 0    ;
         0, cos(a) , sin(a) ;
         0, -sin(a), cos(a) ];
     
T_pitch = [cos(b),0,-sin(b) ;
        0     ,1,0       ;
        sin(b),0,cos(b)  ];
    
T_yaw = [cos(c) ,sin(c),0;
        -sin(c),cos(c),0;
        0      ,0     ,1];

T_BE = T_roll * T_pitch * T_yaw;

V_e = T_BE^-1 * [u;v;w];

u_e = V_e(1);
v_e = V_e(2);
w_e = V_e(3);

u_b = u;
v_b = v;
w_b = w;
